simulink model "inital"  (Simulink 10.0)
settings: Solver=ode45  StartTime=0.0  StopTime=10.0  RelTol=1e-3  EnableMultiTasking=on
settings Model: Creator=bhisma  LastModifiedBy=bhisma
settings DataIOCC: LimitDataPoints=on  SignalLoggingSaveFormat=ModelDataLogs
settings OptimizationCC: BlockReduction=off  BooleanDataType=off  LifeSpan=auto
settings DebuggingCC: SaveWithParameterizedLinksMsg=none  SignalResolutionControl=TryResolveAllWithWarning  MultiTaskDSMMsg=warning  MultiTaskCondExecSysMsg=none  SFUnexpectedBacktrackingDiag=error  SFNoUnconditionalDefaultTransitionDiag=error  SFExecutionAtInitializationDiag=warning  ArithmeticOperatorsInVariantConditions=error
settings HardwareCC: ProdBitPerPointer=64  ProdBitPerSizeT=64  ProdBitPerPtrDiffT=64  ProdLargestAtomicFloat=Float  ProdIntDivRoundTo=Zero  ProdEndianess=LittleEndian  ProdWordSize=64  ProdHWDeviceType=Intel->x86-64 (Windows64)  TargetUnknown=on
settings SFSimCC: SimUseLocalCustomCode=on  CustomCodeUndefinedFunction=FilterOut
settings RTWCC: RTWUseLocalCustomCode=on
settings CodeAppCC: StateflowObjectComments=off
settings GRTTargetCC: TargetLangStandard=C99 (ISO)
settings ConfigComp: CovMetricSettings=dwe  CovSaveCumulativeToWorkspaceVar=off  CovSaveSingleToWorkspaceVar=off

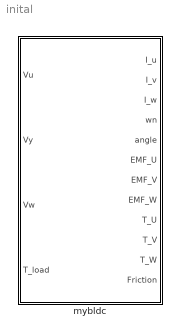
== system inital ==
  mybldc : Subsystem

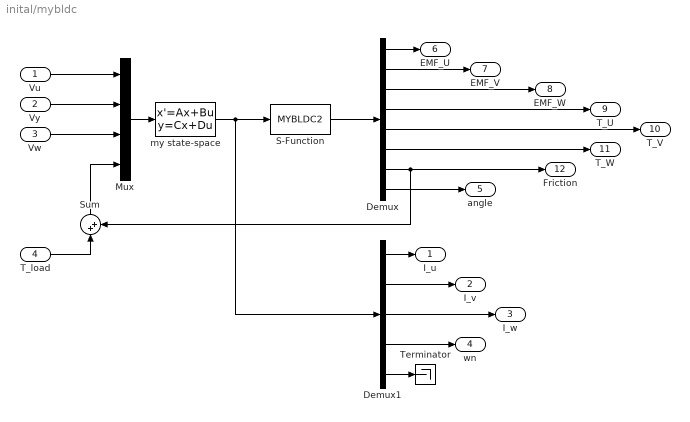
== system inital/mybldc ==
  Vu : Inport
  Vy : Inport  Port=2
  Vw : Inport  Port=3
  T_load : Inport  Port=4
  Demux : Demux  Outputs=8
  Demux1 : Demux  Outputs=5
  Mux : Mux
  S-Function : S-Function  FunctionName=MYBLDC2  Parameters=N,R,L,M,BM,Rl,Rr,DF,J,P,F0,Fs  SFunctionDeploymentMode=off  EnableBusSupport=off  mask{N=100, R=0.7, L=2.72e-3, M=-1.5e-3, BM=49/60, Rl=0.03, Rr=0.02, DF=0.002, J=0.0002, P=4, Fs=0.2*0.089, F0=0.089}
      mask prompts: N "Number of turns per phase"; R "Resistance per phase"; L "self inductance per phase"; M "mutual inductace per phase"; BM "Maximum value of flux density"; Rl "Rotor length"; Rr "rotor radius"; DF "value of viscous friction"; J "moment of inertia"; P "Total number of poles"; Fs "starting value of coulomb friction"; F0 "Static friction"
  Sum : Sum  Inputs=|++  SaturateOnIntegerOverflow=on  InputSameDT=on  OutDataTypeStr=Inherit: Same as first input
  Terminator : Terminator
  my state-space : StateSpace  A="[ -1.658768e+002  0 0 0 0; 0  -1.658768e+002 0 1.161137e+001 0; 0  0 -1.658768e+002 -1.161137e+001 0; 0  -245 245 -10 0; 0  0 0 2 0]"  B=[236.96 0 0 0; 0 236.96 0 0; 0 0 236.96 0; 0 0 0 -5000; 0 0 0 0]  C=[1 0 0 0 0;0 1 0 0 0;0 0 1 0 0; 0 0 0 1 0;0 0 0 0 1]  D=[0 0 0 0 ; 0 0 0 0; 0 0 0 0; 0 0 0 0; 0 0 0 0]  InitialCondition=[0 0 0 0 0]
  I_u : Outport
  I_v : Outport  Port=2
  I_w : Outport  Port=3
  wn : Outport  Port=4
  angle : Outport  Port=5
  EMF_U : Outport  Port=6
  EMF_V : Outport  Port=7
  EMF_W : Outport  Port=8
  T_U : Outport  Port=9
  T_V : Outport  Port=10
  T_W : Outport  Port=11
  Friction : Outport  Port=12
  wires:
  Vw/1 -> Mux/3
  Vy/1 -> Mux/2
  Vu/1 -> Mux/1
  Mux/1 -> my state-space/1
  my state-space/1 -> S-Function/1, Demux1/1
  S-Function/1 -> Demux/1
  Demux1/1 -> I_u/1
  Demux/1 -> EMF_U/1
  Demux/2 -> EMF_V/1
  Demux/3 -> EMF_W/1
  Demux/4 -> T_U/1
  Demux/5 -> T_V/1
  Demux/6 -> T_W/1
  Demux/7 -> Friction/1, Sum/2
  Demux/8 -> angle/1
  Demux1/2 -> I_v/1
  Demux1/3 -> I_w/1
  Demux1/4 -> wn/1
  Demux1/5 -> Terminator/1
  Sum/1 -> Mux/4
  T_load/1 -> Sum/1
